simulink model "bh_smd_MAIN"  (R2018a)
settings: Solver=ode45  StartTime=0.0  StopTime=10.0  RelTol=1e-7
undefined symbols (not defined in the file): c, k, m, x_init, xdot_init
settings Model: Creator=bhorton  LastModifiedBy=bhorton
settings CodeAppCC: StateflowObjectComments=on

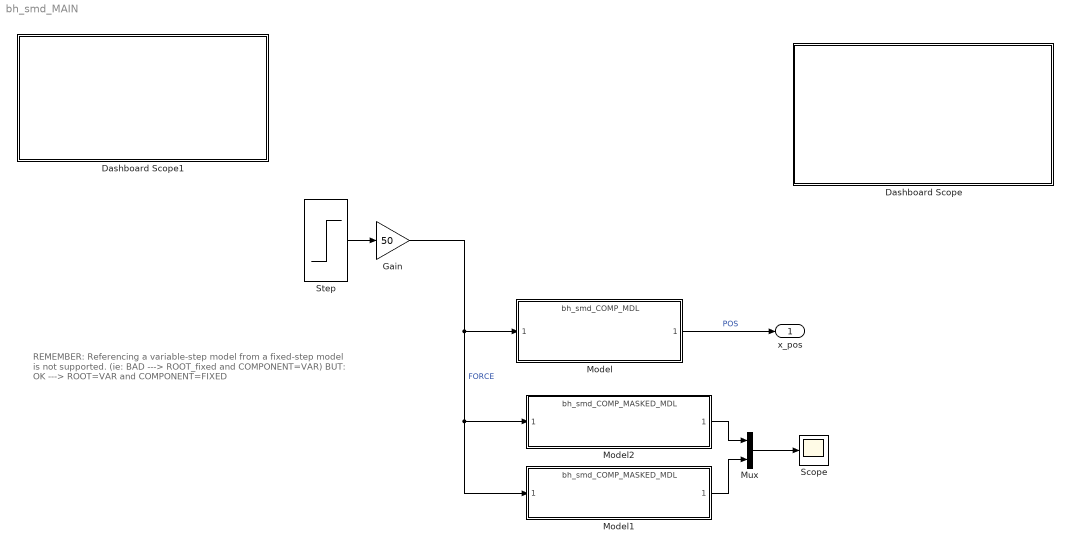
== system bh_smd_MAIN ==
  note: REMEMBER:
      |
      | Referencing a variable-step model
      | from a fixed-step model is not supported.
      | (ie: BAD ---> ROOT_fixed and COMPONENT=VAR)
      |
      | BUT:
      | OK ---> ROOT=VAR and COMPONENT=FIXED
  Dashboard Scope : Subsystem  DialogController=hmiCreateDDGDialog  IsWebBlock=on  mask(MWDashboardBlock){webBlockId=47d7a76a-e090-4f37-bb13-c45fee118520, webBlockType=sdiscope, ShowInitialText=on, HMISrcModelName=bh_smd_MAIN}
      mask prompts: webBlockId "WebBlock Id"; webBlockType "WebBlock Type"; HMISrcModelName "Source Model"
      mask help: SimulinkHMI:dialogs:HMIScopeDialogDesc
      mask Help: helpview([docroot '/mapfiles/simulink.map'], 'hmi_scope')
      mask Display:
      | if strcmp(get_param(bdroot(gcb),'BlockDiagramType'), 'library')
      |     image([(matlabroot) '/toolbox/simulink/hmi/icons/DashboardScope.png']);
      | end
  Dashboard Scope1 : Subsystem  DialogController=hmiCreateDDGDialog  IsWebBlock=on  mask(MWDashboardBlock){webBlockId=8ddedbd7-6b40-4d71-b8ad-862d34055e22, webBlockType=sdiscope, ShowInitialText=on, HMISrcModelName=bh_smd_MAIN}
      mask prompts: webBlockId "WebBlock Id"; webBlockType "WebBlock Type"; HMISrcModelName "Source Model"
      mask help: SimulinkHMI:dialogs:HMIScopeDialogDesc
      mask Help: helpview([docroot '/mapfiles/simulink.map'], 'hmi_scope')
      mask Display:
      | if strcmp(get_param(bdroot(gcb),'BlockDiagramType'), 'library')
      |     image([(matlabroot) '/toolbox/simulink/hmi/icons/DashboardScope.png']);
      | end
  Gain : Gain  Gain=50
  Model : ModelReference  ModelNameDialog=bh_smd_COMP_MDL.slx  SimulationMode=Normal  ModelReferenceVersion=1.40
  Model1 : ModelReference  ModelNameDialog=bh_smd_COMP_MASKED_MDL.slx  ParameterArgumentNames=c,k,m,x_init,xdot_init  ParameterArgumentValues=c,k,m,x_init,xdot_init  UsingDefaultArgumentValue=0,0,0,0,0  SimulationMode=Normal  ModelReferenceVersion=1.43  m=m  c=c/2  k=k  x_init=5  xdot_init=0  SimulationMode=Normal
  Model2 : ModelReference  ModelNameDialog=bh_smd_COMP_MASKED_MDL.slx  ParameterArgumentNames=c,k,m,x_init,xdot_init  ParameterArgumentValues=c,k,m,x_init,xdot_init  UsingDefaultArgumentValue=0,0,0,0,0  SimulationMode=Normal  ModelReferenceVersion=1.43  m=m  c=c  k=k  x_init=5  xdot_init=0  SimulationMode=Normal
  Mux : Mux  Inputs=2
  Scope : Scope
  Step : Step  Time=5  SampleTime=0
  x_pos : Outport
  wires:
  Step/1 -> Gain/1
  Gain/1 -> Model2/1, Model1/1, Model/1  "FORCE"
  Model/1 -> x_pos/1  "POS"
  Mux/1 -> Scope/1
  Model1/1 -> Mux/2
  Model2/1 -> Mux/1

== system bh_smd_MAIN/Dashboard Scope ==

== system bh_smd_MAIN/Dashboard Scope1 ==
